simulink model "Tanques"  (R2021a)
settings: Solver=VariableStepAuto  StartTime=0.0  StopTime=40.0  RelTol=1e-3
settings Model: Creator=Santiago  LastModifiedBy=Santiago

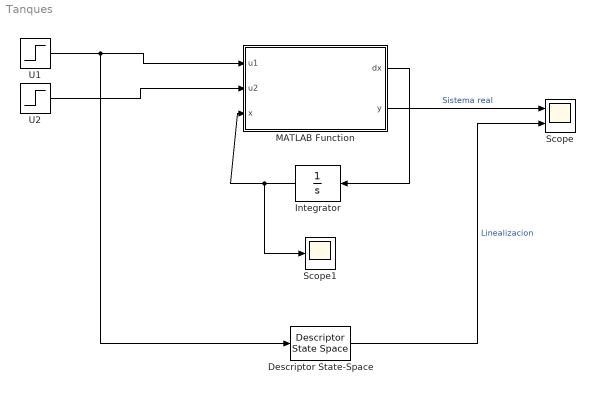
== system Tanques ==
  Descriptor State-Space : DescriptorStateSpace  E=[1 0; 0 1]  A=[-0.5 0.5; 0.5 -1]  B=[1; 0]  C=[0 0.5]  D=0  DirectFeedthrough=Auto
  Integrator : Integrator
  MATLAB Function : MATLAB Function  TreatAsAtomicUnit=on
  Scope : Scope  NumInputPorts=2
  Scope1 : Scope
  U1 : Step  SampleTime=0
  U2 : Step  After=0  SampleTime=0
  wires:
  MATLAB Function/1(dx) -> Integrator/1
  Integrator/1 -> Scope1/1, MATLAB Function/3(x)
  MATLAB Function/2(y) -> Scope/1  "Sistema real"
  U2/1 -> MATLAB Function/2(u2)
  U1/1 -> Descriptor State-Space/1, MATLAB Function/1(u1)
  Descriptor State-Space/1 -> Scope/2  "Linealizacion"

== matlab function Tanques/MATLAB Function ==
  data: u1 input; dx output size=[2, 1]; u2 input; x input; y output
function [dx, y] = sys(u1, u2, x)

dx = zeros(2, 1);

y = sqrt(abs(x(2)))

dx(1) = -sqrt(abs(x(1) - x(2))) + u1
dx(2) = sqrt(abs(x(1) - x(2))) - sqrt(abs(x(2))) + u2
%nota: puse abs() porque a veces aparecían números negativos en las raíces
%(por errores numéricos)
;
